simulink model "newEMB"  (R2023a)
settings: Solver=FixedStepAuto  StartTime=0.0  StopTime=5  FixedStep=5e-5  RelTol=1e-3
model workspace (MAT data in the model file):
  Bv = 0.001086
  L = 0.005
  Tc = 0.0192
  Ts = 0.0387
  Ws = 1
  deta = 1
  ng = 0.9
  ns = 0.9
libraries: slpidlib x3, spsDCVoltageSourceLib x1, spsPermanentMagnetSynchronousMachineLib x1, spsSVPWMGenerator2LevelLib x1, spsUniversalBridgeLib x1, spsabctodq0Lib x1, sps_lib x1, spsdq0toAlphaBetaZeroLib x1
settings Model: Creator=ASUS  LastModifiedBy=13524
settings SolverCC: AlgebraicLoopSolver=TrustRegion
settings DataIOCC: ReturnWorkspaceOutputs=off
settings DebuggingCC: UnconnectedInputMsg=warning  UnconnectedOutputMsg=warning  UnconnectedLineMsg=warning  ArithmeticOperatorsInVariantConditions=warning
settings ModelReferenceCC: EnableRefExpFcnMdlSchedulingChecks=on
settings SFSimCC: SimUseLocalCustomCode=off  CustomCodeUndefinedFunction=UseInterfaceOnly
settings RTWCC: RTWUseLocalCustomCode=off

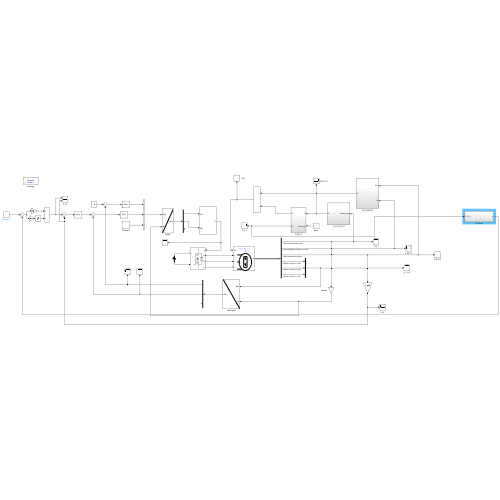
[thumbnail: Simulink's stored preview of the top-level diagram]
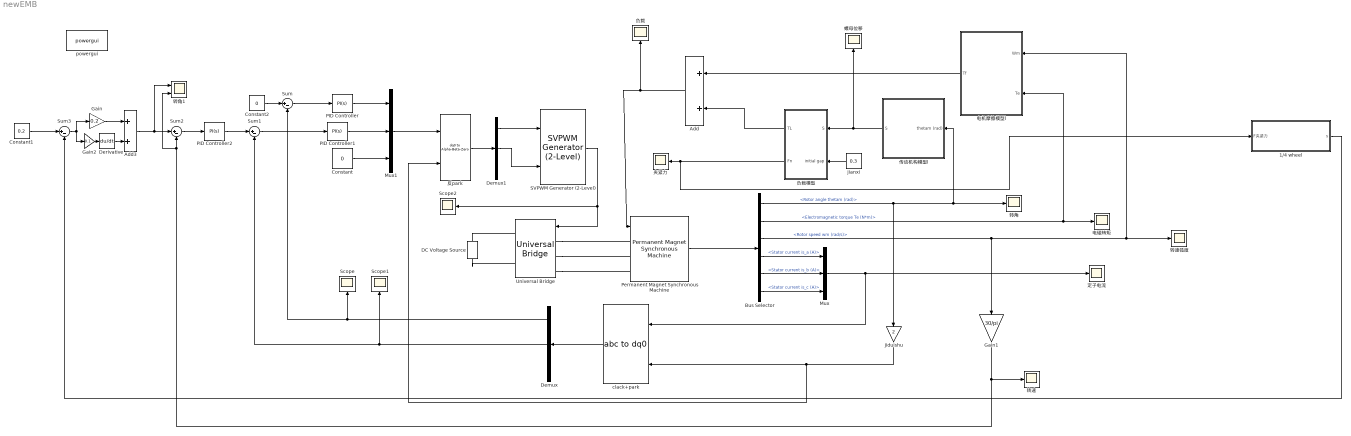
== system newEMB ==
  1/4 wheel : Subsystem
  Add : Sum
  Add3 : Sum
  Bus Selector : BusSelector  OutputSignals=Rotor angle thetam (rad),Electromagnetic torque Te (N*m),Rotor speed wm (rad/s),Stator current is_a (A),Stator current is_b (A),Stator current is_c (A)
  Constant : Constant  Value=0  VectorParams1D=off  SampleTime=-1
  Constant1 : Constant  Value=0.2
  Constant2 : Constant  Value=0
  DC Voltage Source : spsDCVoltageSourceLib/DC Voltage Source  Amplitude=60  Measurements=None
  Demux : Demux  Outputs=3
  Demux1 : Demux  Outputs=3
  Derivative : Derivative
  Gain : Gain  Gain=0.2
  Gain1 : Gain  Gain=30/pi
  Gain2 : Gain  Gain=0.1
  Mux : Mux  Inputs=3
  Mux1 : Mux  Inputs=3
  PID Controller : slpidlib/PID Controller  Controller=PI  Form=Parallel  TimeDomain=Continuous-time  UseExternalTs=off  SampleTime=-1  IntegratorMethod=Forward Euler  FilterMethod=Forward Euler  ControllerParametersSource=internal  P=1  I=1  UseKiTs=off  D=0  N=100  UseFilter=on  TunerSelectOption=Transfer Function Based (PID Tuner App)  InitialConditionSource=internal  InitialConditionForIntegrator=0  InitialConditionForFilter=0  DifferentiatorICPrevScaledInput=0  ExternalReset=none  TrackingMode=off  Kt=1  LimitOutput=off  SatLimitsSource=internal  UpperSaturationLimit=inf  LowerSaturationLimit=-inf  LinearizeAsGain=on  AntiWindupMode=none  Kb=1  LimitIntegrator=off  UpperIntegratorSaturationLimit=inf  LowerIntegratorSaturationLimit=-inf  POutMin=[]  POutMax=[]  IOutMin=[]  IOutMax=[]  DOutMin=[]  DOutMax=[]  NOutMin=[]  NOutMax=[]  SumOutMin=[]  SumOutMax=[]  SaturationOutMin=[]  SaturationOutMax=[]  PParamMin=[]  PParamMax=[]  IParamMin=[]  IParamMax=[]  DParamMin=[]  DParamMax=[]  NParamMin=[]  NParamMax=[]  KbParamMin=[]  KbParamMax=[]  KtParamMin=[]  KtParamMax=[]  KbOutMin=[]  KbOutMax=[]  KtOutMin=[]  KtOutMax=[]  IntegratorOutMin=[]  IntegratorOutMax=[]  FilterOutMin=[]  FilterOutMax=[]  SumI1OutMin=[]  SumI1OutMax=[]  SumI2OutMin=[]  SumI2OutMax=[]  SumI3OutMin=[]  SumI3OutMax=[]  SumI4OutMin=[]  SumI4OutMax=[]  SumDOutMin=[]  SumDOutMax=[]  DifferentiatorOutMin=[]  DifferentiatorOutMax=[]  FilterDiffOutCoefMin=[]  FilterDiffOutCoefMax=[]  ReciprocalOutMin=[]  ReciprocalOutMax=[]  SumDenOutMin=[]  SumDenOutMax=[]  SumNumOutMin=[]  SumNumOutMax=[]  DivideOutMin=[]  DivideOutMax=[]  UdiffTsProdOutMin=[]  UdiffTsProdOutMax=[]  NTsProdOutMin=[]  NTsProdOutMax=[]  UintegralTsProdOutMin=[]  UintegralTsProdOutMax=[]  UngainTsProdOutMin=[]  UngainTsProdOutMax=[]  ClampingZeroOutDataTypeStr=Inherit: Inherit via back propagation  ClampingZeroOutMin=[]  ClampingZeroOutMax=[]  FilterDenConstantOutDataTypeStr=Inherit: Inherit via back propagation  FilterDenConstantOutMin=[]  FilterDenConstantOutMax=[]  PCopyOutDataTypeStr=Inherit: Inherit via back propagation  PCopyOutMin=[]  PCopyOutMax=[]  NCopyOutDataTypeStr=Inherit: Inherit via back propagation  NCopyOutMin=[]  NCopyOutMax=[]  IntegratorContinuousStateAttributes=''  IntegratorStateMustResolveToSignalObject=off  IntegratorRTWStateStorageClass=Auto  FilterContinuousStateAttributes=''  FilterStateMustResolveToSignalObject=off  FilterRTWStateStorageClass=Auto  ParallelPVariant=InternalParameters  IdealPVariant=Disabled  IVariant=InternalParameters  DVariant=Disabled  IntegratorVariant=Continuous  SatVariant=Disabled  AWVariant=Passthrough  PCopyVariant=Disabled  TRVariant=Disabled  FdbkBlocksVariant=Forward  IdealPFdbkVariant=Disabled  SatFdbkVariant=Disabled  DerivativeFilterVariant=Disabled  NVariant=Disabled  NCopyVariant=Disabled_SignalSpec  FilterICVariant=Disabled  IntegratorICVariant=InternalICs  ExternalResetVariant=Disabled  TRSumVariant=Passthrough  SumFdbkVariant=Disabled  SumVariant=Sum_PI  TsampFilterVariant=InternalTs  TsampNgainVariant=Passthrough  TsampIntegralVariant=Disabled_SignalSpec  ExternalSaturationOutDataTypeStr=Inherit: Same as second input
  PID Controller1 : slpidlib/PID Controller  Controller=PI  Form=Parallel  TimeDomain=Continuous-time  UseExternalTs=off  SampleTime=-1  IntegratorMethod=Forward Euler  FilterMethod=Forward Euler  ControllerParametersSource=internal  P=1  I=1  UseKiTs=off  D=0  N=100  UseFilter=on  TunerSelectOption=Transfer Function Based (PID Tuner App)  InitialConditionSource=internal  InitialConditionForIntegrator=0  InitialConditionForFilter=0  DifferentiatorICPrevScaledInput=0  ExternalReset=none  TrackingMode=off  Kt=1  LimitOutput=off  SatLimitsSource=internal  UpperSaturationLimit=inf  LowerSaturationLimit=-inf  LinearizeAsGain=on  AntiWindupMode=none  Kb=1  LimitIntegrator=off  UpperIntegratorSaturationLimit=inf  LowerIntegratorSaturationLimit=-inf  POutMin=[]  POutMax=[]  IOutMin=[]  IOutMax=[]  DOutMin=[]  DOutMax=[]  NOutMin=[]  NOutMax=[]  SumOutMin=[]  SumOutMax=[]  SaturationOutMin=[]  SaturationOutMax=[]  PParamMin=[]  PParamMax=[]  IParamMin=[]  IParamMax=[]  DParamMin=[]  DParamMax=[]  NParamMin=[]  NParamMax=[]  KbParamMin=[]  KbParamMax=[]  KtParamMin=[]  KtParamMax=[]  KbOutMin=[]  KbOutMax=[]  KtOutMin=[]  KtOutMax=[]  IntegratorOutMin=[]  IntegratorOutMax=[]  FilterOutMin=[]  FilterOutMax=[]  SumI1OutMin=[]  SumI1OutMax=[]  SumI2OutMin=[]  SumI2OutMax=[]  SumI3OutMin=[]  SumI3OutMax=[]  SumI4OutMin=[]  SumI4OutMax=[]  SumDOutMin=[]  SumDOutMax=[]  DifferentiatorOutMin=[]  DifferentiatorOutMax=[]  FilterDiffOutCoefMin=[]  FilterDiffOutCoefMax=[]  ReciprocalOutMin=[]  ReciprocalOutMax=[]  SumDenOutMin=[]  SumDenOutMax=[]  SumNumOutMin=[]  SumNumOutMax=[]  DivideOutMin=[]  DivideOutMax=[]  UdiffTsProdOutMin=[]  UdiffTsProdOutMax=[]  NTsProdOutMin=[]  NTsProdOutMax=[]  UintegralTsProdOutMin=[]  UintegralTsProdOutMax=[]  UngainTsProdOutMin=[]  UngainTsProdOutMax=[]  ClampingZeroOutDataTypeStr=Inherit: Inherit via back propagation  ClampingZeroOutMin=[]  ClampingZeroOutMax=[]  FilterDenConstantOutDataTypeStr=Inherit: Inherit via back propagation  FilterDenConstantOutMin=[]  FilterDenConstantOutMax=[]  PCopyOutDataTypeStr=Inherit: Inherit via back propagation  PCopyOutMin=[]  PCopyOutMax=[]  NCopyOutDataTypeStr=Inherit: Inherit via back propagation  NCopyOutMin=[]  NCopyOutMax=[]  IntegratorContinuousStateAttributes=''  IntegratorStateMustResolveToSignalObject=off  IntegratorRTWStateStorageClass=Auto  FilterContinuousStateAttributes=''  FilterStateMustResolveToSignalObject=off  FilterRTWStateStorageClass=Auto  ParallelPVariant=InternalParameters  IdealPVariant=Disabled  IVariant=InternalParameters  DVariant=Disabled  IntegratorVariant=Continuous  SatVariant=Disabled  AWVariant=Passthrough  PCopyVariant=Disabled  TRVariant=Disabled  FdbkBlocksVariant=Forward  IdealPFdbkVariant=Disabled  SatFdbkVariant=Disabled  DerivativeFilterVariant=Disabled  NVariant=Disabled  NCopyVariant=Disabled_SignalSpec  FilterICVariant=Disabled  IntegratorICVariant=InternalICs  ExternalResetVariant=Disabled  TRSumVariant=Passthrough  SumFdbkVariant=Disabled  SumVariant=Sum_PI  TsampFilterVariant=InternalTs  TsampNgainVariant=Passthrough  TsampIntegralVariant=Disabled_SignalSpec  ExternalSaturationOutDataTypeStr=Inherit: Same as second input
  PID Controller2 : slpidlib/PID Controller  Controller=PI  Form=Parallel  TimeDomain=Continuous-time  UseExternalTs=off  SampleTime=-1  IntegratorMethod=Forward Euler  FilterMethod=Forward Euler  ControllerParametersSource=internal  P=1  I=1  UseKiTs=off  D=0  N=100  UseFilter=on  TunerSelectOption=Transfer Function Based (PID Tuner App)  InitialConditionSource=internal  InitialConditionForIntegrator=0  InitialConditionForFilter=0  DifferentiatorICPrevScaledInput=0  ExternalReset=none  TrackingMode=off  Kt=1  LimitOutput=off  SatLimitsSource=internal  UpperSaturationLimit=inf  LowerSaturationLimit=-inf  LinearizeAsGain=on  AntiWindupMode=none  Kb=1  LimitIntegrator=off  UpperIntegratorSaturationLimit=inf  LowerIntegratorSaturationLimit=-inf  POutMin=[]  POutMax=[]  IOutMin=[]  IOutMax=[]  DOutMin=[]  DOutMax=[]  NOutMin=[]  NOutMax=[]  SumOutMin=[]  SumOutMax=[]  SaturationOutMin=[]  SaturationOutMax=[]  PParamMin=[]  PParamMax=[]  IParamMin=[]  IParamMax=[]  DParamMin=[]  DParamMax=[]  NParamMin=[]  NParamMax=[]  KbParamMin=[]  KbParamMax=[]  KtParamMin=[]  KtParamMax=[]  KbOutMin=[]  KbOutMax=[]  KtOutMin=[]  KtOutMax=[]  IntegratorOutMin=[]  IntegratorOutMax=[]  FilterOutMin=[]  FilterOutMax=[]  SumI1OutMin=[]  SumI1OutMax=[]  SumI2OutMin=[]  SumI2OutMax=[]  SumI3OutMin=[]  SumI3OutMax=[]  SumI4OutMin=[]  SumI4OutMax=[]  SumDOutMin=[]  SumDOutMax=[]  DifferentiatorOutMin=[]  DifferentiatorOutMax=[]  FilterDiffOutCoefMin=[]  FilterDiffOutCoefMax=[]  ReciprocalOutMin=[]  ReciprocalOutMax=[]  SumDenOutMin=[]  SumDenOutMax=[]  SumNumOutMin=[]  SumNumOutMax=[]  DivideOutMin=[]  DivideOutMax=[]  UdiffTsProdOutMin=[]  UdiffTsProdOutMax=[]  NTsProdOutMin=[]  NTsProdOutMax=[]  UintegralTsProdOutMin=[]  UintegralTsProdOutMax=[]  UngainTsProdOutMin=[]  UngainTsProdOutMax=[]  ClampingZeroOutDataTypeStr=Inherit: Inherit via back propagation  ClampingZeroOutMin=[]  ClampingZeroOutMax=[]  FilterDenConstantOutDataTypeStr=Inherit: Inherit via back propagation  FilterDenConstantOutMin=[]  FilterDenConstantOutMax=[]  PCopyOutDataTypeStr=Inherit: Inherit via back propagation  PCopyOutMin=[]  PCopyOutMax=[]  NCopyOutDataTypeStr=Inherit: Inherit via back propagation  NCopyOutMin=[]  NCopyOutMax=[]  IntegratorContinuousStateAttributes=''  IntegratorStateMustResolveToSignalObject=off  IntegratorRTWStateStorageClass=Auto  FilterContinuousStateAttributes=''  FilterStateMustResolveToSignalObject=off  FilterRTWStateStorageClass=Auto  ParallelPVariant=InternalParameters  IdealPVariant=Disabled  IVariant=InternalParameters  DVariant=Disabled  IntegratorVariant=Continuous  SatVariant=Disabled  AWVariant=Passthrough  PCopyVariant=Disabled  TRVariant=Disabled  FdbkBlocksVariant=Forward  IdealPFdbkVariant=Disabled  SatFdbkVariant=Disabled  DerivativeFilterVariant=Disabled  NVariant=Disabled  NCopyVariant=Disabled_SignalSpec  FilterICVariant=Disabled  IntegratorICVariant=InternalICs  ExternalResetVariant=Disabled  TRSumVariant=Passthrough  SumFdbkVariant=Disabled  SumVariant=Sum_PI  TsampFilterVariant=InternalTs  TsampNgainVariant=Passthrough  TsampIntegralVariant=Disabled_SignalSpec  ExternalSaturationOutDataTypeStr=Inherit: Same as second input
  Permanent Magnet Synchronous Machine : spsPermanentMagnetSynchronousMachineLib/Permanent Magnet Synchronous Machine  NbPhases=3  FluxDistribution=Sinusoidal  RotorType=Round  MechanicalLoad=Torque Tm  PresetModel=No  ShowDetailedParameters=on  MeasurementBus=off  Resistance=0.57  Inductance=8.5e-3  dqInductances=[8.5e-3,8.5e-3]  La=0.000625  MachineConstant=Flux linkage established by magnets (V.s)  Flux=0.0155  VoltageCst=5.6228  TorqueCst=0.0465  Flat=120  Mechanical=[0.0000342 0.0002024 2 0]  PolePairs=4  InitialConditions=[0,0, 0,0]  InitialConditions5ph=[0 0 0 0 0 0]  RefAngle=90 degrees behind phase A axis (modified Park)  IterativeDiscreteModel=Trapezoidal non iterative  TsBlock=-1  TsPowergui=0
  SVPWM Generator (2-Level) : spsSVPWMGenerator2LevelLib/SVPWM Generator (2-Level)  InputType=alpha-beta components  SwitchingPattern=Pattern #1  Fc=2000  ParUref=[0.8 -30 50]  Ts=0
  Scope : Scope
  Scope1 : Scope
  Scope2 : Scope
  Sum{,1..3} (4 alike) : Sum  Inputs=|+-
  Universal Bridge : spsUniversalBridgeLib/Universal Bridge  Arms=3  SnubberResistance=1e5  SnubberCapacitance=inf  Device=MOSFET / Diodes  Ron=1e-3  Lon=0  ForwardVoltages="[  0  0  ]"  ForwardVoltage=0  GTOparameters=[ 10e-6 , 20e-6 ]  IGBTparameters=[ 1e-6 , 2e-6 ]  Measurements=None  Measurements_2=None  converterType=Rectifier
  clack+park : spsabctodq0Lib/abc to dq0  Alignment=90 degrees behind phase A axis
  jianxi : Constant  Value=0.3
  jiduishu : Gain  Gain=2
  powergui : sps_lib/powergui  Priority=1  SimulationMode=Discrete  SampleTime=5e-5  frequency=60  Iterations=50  frequencyindice=0  Pbase=100e6  ErrMax=1e-4  UnitsV=kV  UnitsW=MW  buscounter=0  FunctionMessages=off  echomessages=off  EnableUseOfTLC=off  CurrentSourceSwitches=off  DisableSnubberDevices=off  DisableRonSwitches=off  DisableVfSwitches=off  DisplayEquations=off  AutomaticDiscreteSolvers=off  SolverType=Tustin/Backward Euler (TBE)  Interpol=off  ExternalGateDelay=off  methode=off  Ts=100  x0status=blocks  SPID=on  SwTol=0  HookPort=off  NonlinearTolerance=1e-4  nMaxIteration=100  ContinueOnMaxIteration=off  RestoreLinks=warning  ResistiveCurrentMeasurement=off  Frange=[0:2:500]  Ylog=off  Xlog=on  ShowGrid=off  save=off  variable=ZData  structure=0  ZoomFFT=off  StartTime=0.0  cycles=1  DisplayStyle=1  fundamental=60  FreqAxis=off  MaxFrequency=1000  frequencyindicesteady=1  RmsSteady=1  display=off
  传动机构模型l : Subsystem
  反park : spsdq0toAlphaBetaZeroLib/dq0 to Alpha-Beta-Zero  Alignment=90 degrees behind phase A axis
  夹紧力 : Scope
  定子电流 : Scope
  电机摩擦模型l : Subsystem
  电磁转矩 : Scope
  螺母位移 : Scope
  负载 : Scope
  负载模型 : Subsystem
  转角 : Scope
  转角1 : Scope  NumInputPorts=2
  转速 : Scope
  转速弧度 : Scope
  wires:
  Permanent Magnet Synchronous Machine/1 -> Bus Selector/1
  Add/1 -> 负载/1, Permanent Magnet Synchronous Machine/1
  电机摩擦模型l/1(Tf) -> Add/1
  负载模型/1(TL) -> Add/2
  Bus Selector/1 -> 转角/1, 传动机构模型l/1(" thetam (rad)"), jiduishu/1  "<Rotor angle thetam (rad)>"
  传动机构模型l/1(S) -> 负载模型/1(S), 螺母位移/1
  jianxi/1 -> 负载模型/2(initial gap)
  Bus Selector/3 -> 转速弧度/1, 电机摩擦模型l/1(Wm), Gain1/1  "<Rotor speed wm (rad/s)>"
  Bus Selector/2 -> 电机摩擦模型l/2(Te), 电磁转矩/1  "<Electromagnetic torque Te (N*m)>"
  Bus Selector/4 -> Mux/1  "<Stator current is_a (A)>"
  Bus Selector/5 -> Mux/2  "<Stator current is_b (A)>"
  Bus Selector/6 -> Mux/3  "<Stator current is_c (A)>"
  Mux/1 -> clack+park/1, 定子电流/1
  SVPWM Generator (2-Level)/1 -> Universal Bridge/1, Scope2/1
  Mux1/1 -> 反park/1
  Sum/1 -> PID Controller/1
  PID Controller/1 -> Mux1/1
  PID Controller1/1 -> Mux1/2
  Constant/1 -> Mux1/3
  Sum1/1 -> PID Controller1/1
  clack+park/1 -> Demux/1
  Demux/1 -> Sum/2, Scope/1
  Demux/2 -> Scope1/1, Sum1/2
  jiduishu/1 -> 反park/2, clack+park/2
  PID Controller2/1 -> Sum1/1
  Sum2/1 -> PID Controller2/1
  Gain1/1 -> 转速/1, 转角1/2, Sum2/2
  Sum3/1 -> Gain2/1, Gain/1
  Constant2/1 -> Sum/1
  反park/1 -> Demux1/1
  Demux1/1 -> SVPWM Generator (2-Level)/1
  Demux1/2 -> SVPWM Generator (2-Level)/2
  Constant1/1 -> Sum3/1
  Add3/1 -> 转角1/1, Sum2/1
  负载模型/2(Fn) -> 1/4 wheel/1(F夹紧力), 夹紧力/1
  Derivative/1 -> Add3/2
  Gain/1 -> Add3/1
  Gain2/1 -> Derivative/1
  1/4 wheel/1(s) -> Sum3/2
  connections:
  Universal Bridge/LConn1 -- Permanent Magnet Synchronous Machine/LConn1
  Universal Bridge/LConn2 -- Permanent Magnet Synchronous Machine/LConn2
  Universal Bridge/LConn3 -- Permanent Magnet Synchronous Machine/LConn3
  DC Voltage Source/RConn1 -- Universal Bridge/RConn1
  DC Voltage Source/LConn1 -- Universal Bridge/RConn2

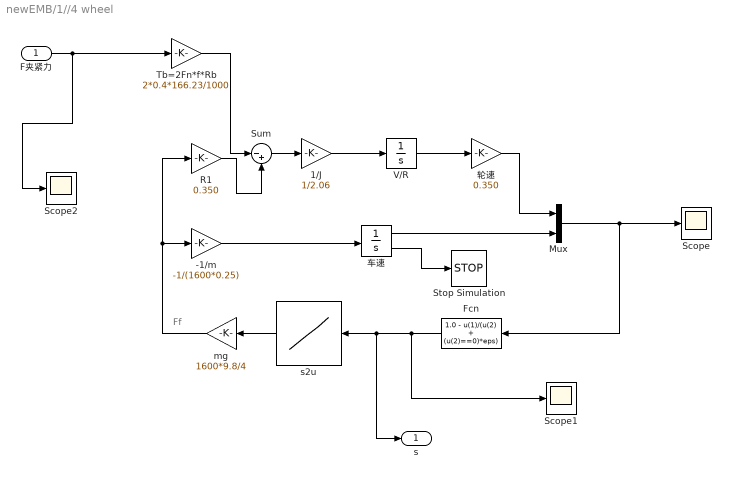
== system newEMB/1//4 wheel ==
  note: Ff
  F夹紧力 : Inport
  -1/m : Gain  Gain=-1/(1600*0.25)
  1/J : Gain  Gain=1/2.06
  Fcn : Fcn  Expr=1.0 - u(1)/(u(2) + (u(2)==0)*eps)
  Mux : Mux  Inputs=2
  R1 : Gain  Gain=0.350
  Scope : Scope
  Scope1 : Scope
  Scope2 : Scope
  Stop Simulation : Stop
  Sum : Sum  Inputs=|-+
  Tb=2Fn*f*Rb : Gain  Gain=2*0.4*166.23/1000
  V/R : Integrator  InitialCondition=40/0.350  LimitOutput=on  UpperSaturationLimit=1000  LowerSaturationLimit=0
  mg : Gain  Gain=1600*9.8/4
  s2u : Lookup_n-D  NumberOfTableDimensions=1  BreakpointsForDimension1=[0;0.05;0.1;0.15;0.2;0.25;0.3;0.35;0.4;0.45;0.5;0.55;0.6;0.65;0.7;0.75;0.8;0.85;0.9;0.95;1]  Table=[0;0.4;0.8;0.97;1;0.98;0.96;0.94;0.92;0.9;0.88;0.855;0.83;0.81;0.79;0.77;0.75;0.73;0.72;0.71;0.7]  InternalRulePriority=Speed  RndMeth=Simplest
  车速 : Integrator  InitialCondition=40  LimitOutput=on  UpperSaturationLimit=100  LowerSaturationLimit=0  ShowSaturationPort=on
  轮速 : Gain  Gain=0.350
  s : Outport
  wires:
  V/R/1 -> 轮速/1
  轮速/1 -> Mux/1
  车速/1 -> Mux/2
  Mux/1 -> Scope/1, Fcn/1
  Fcn/1 -> Scope1/1, s/1, s2u/1
  s2u/1 -> mg/1
  -1/m/1 -> 车速/1
  mg/1 -> R1/1, -1/m/1
  R1/1 -> Sum/2
  Sum/1 -> 1/J/1
  车速/2 -> Stop Simulation/1
  1/J/1 -> V/R/1
  F夹紧力/1 -> Scope2/1, Tb=2Fn*f*Rb/1
  Tb=2Fn*f*Rb/1 -> Sum/1

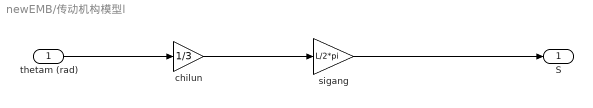
== system newEMB/传动机构模型l ==
  " thetam (rad)" : Inport
  chilun : Gain  Gain=1/3
  sigang : Gain  Gain=L/2*pi
  S : Outport  VectorParamsAs1DForOutWhenUnconnected=off
  wires:
  chilun/1 -> sigang/1
  sigang/1 -> S/1
  " thetam (rad)"/1 -> chilun/1

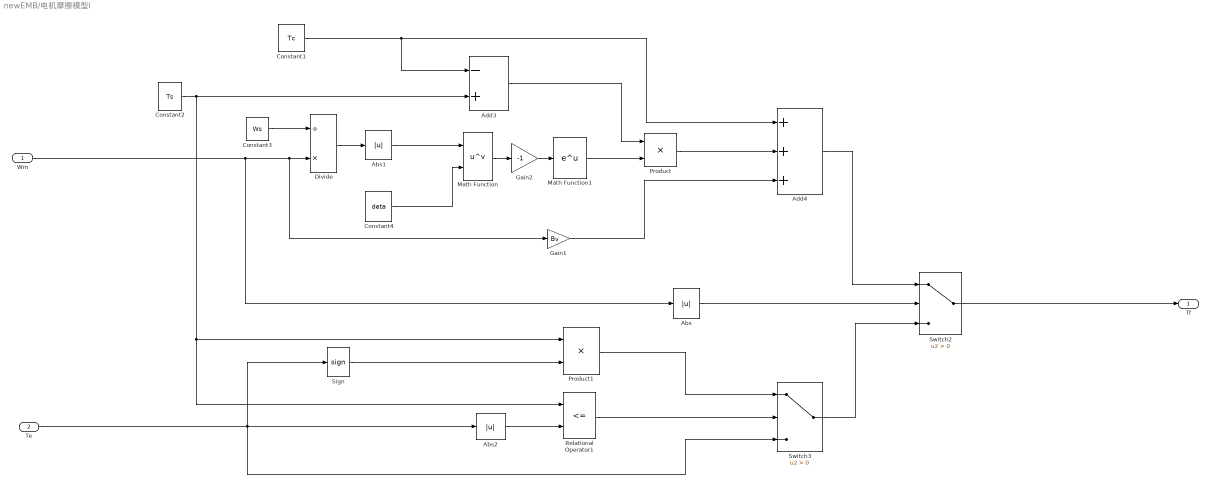
== system newEMB/电机摩擦模型l ==
  Wm : Inport
  Te : Inport  Port=2
  Abs : Abs  SaturateOnIntegerOverflow=off
  Abs1 : Abs  SaturateOnIntegerOverflow=off
  Abs2 : Abs  SaturateOnIntegerOverflow=off
  Add3 : Sum  Inputs=-+
  Add4 : Sum  Inputs=+++
  Constant1 : Constant  Value=Tc
  Constant2 : Constant  Value=Ts
  Constant3 : Constant  Value=Ws
  Constant4 : Constant  Value=deta
  Divide : Product  Inputs=/*
  Gain1 : Gain  Gain=Bv
  Gain2 : Gain  Gain=-1
  Math Function : Math  Operator=pow  SignedPower=on
  Math Function1 : Math  SignedPower=on
  Product : Product
  Product1 : Product
  Relational Operator1 : RelationalOperator  Operator=<=  OutDataTypeStr=boolean  RndMeth=Simplest  InputSameDT=off
  Sign : Signum
  Switch2 : Switch  Criteria=u2 > Threshold  SaturateOnIntegerOverflow=off  InputSameDT=off
  Switch3 : Switch  Criteria=u2 > Threshold  SaturateOnIntegerOverflow=off  InputSameDT=off
  Tf : Outport  VectorParamsAs1DForOutWhenUnconnected=off
  wires:
  Math Function1/1 -> Product/2
  Wm/1 -> Abs/1, Gain1/1, Divide/2
  Abs1/1 -> Math Function/1
  Add4/1 -> Switch2/1
  Gain1/1 -> Add4/3
  Constant4/1 -> Math Function/2
  Te/1 -> Switch3/3, Abs2/1, Sign/1
  Switch3/1 -> Switch2/3
  Add3/1 -> Product/1
  Gain2/1 -> Math Function1/1
  Constant2/1 -> Add3/2, Relational Operator1/1, Product1/1
  Math Function/1 -> Gain2/1
  Divide/1 -> Abs1/1
  Abs/1 -> Switch2/2
  Constant1/1 -> Add3/1, Add4/1
  Relational Operator1/1 -> Switch3/2
  Sign/1 -> Product1/2
  Product1/1 -> Switch3/1
  Abs2/1 -> Relational Operator1/2
  Constant3/1 -> Divide/1
  Product/1 -> Add4/2
  Switch2/1 -> Tf/1

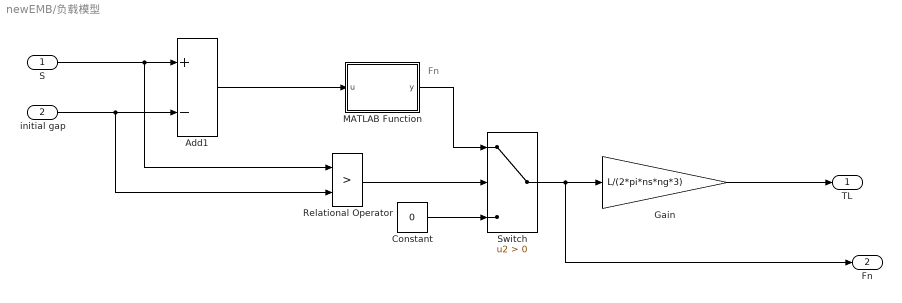
== system newEMB/负载模型 ==
  note: Fn
  S : Inport
  initial gap : Inport  Port=2
  Add1 : Sum  Inputs=+-
  Constant : Constant  Value=0
  Gain : Gain  Gain=L/(2*pi*ns*ng*3)
  MATLAB Function : MATLAB Function  TreatAsAtomicUnit=on
  Relational Operator : RelationalOperator  Operator=>  OutDataTypeStr=boolean  RndMeth=Simplest  InputSameDT=off
  Switch : Switch  Criteria=u2 > Threshold  SaturateOnIntegerOverflow=off  InputSameDT=off
  TL : Outport  VectorParamsAs1DForOutWhenUnconnected=off
  Fn : Outport  Port=2
  wires:
  Switch/1 -> Fn/1, Gain/1
  Gain/1 -> TL/1
  S/1 -> Add1/1, Relational Operator/1
  Relational Operator/1 -> Switch/2
  MATLAB Function/1(y) -> Switch/1
  Constant/1 -> Switch/3
  Add1/1 -> MATLAB Function/1(u)
  initial gap/1 -> Relational Operator/2, Add1/2

== matlab function newEMB/负载模型/MATLAB Function ==
  data: u input; y output
function y = fcn(u)
if u>0.112
   y=-1805*u^3+27290*u^2-6036*u+376.2
else
   y=356.767*u
end
